simulink model "Part_f"  (R2016a)
settings: Solver=VariableStepAuto  StartTime=0.0  StopTime=10.0  RelTol=1e-3
values from neighbouring files (symbols this model uses):
  A = [1,0.00958419619475136,0.0104077383156783,0;0,0.880217654134450,2.02956823954280,0;0,-0.102406711940655,0.862350586928406,0;1,0.00958419619475136,0.0104077383156783,1]    [Project_2.m]
  B = [0.0388811995595289;11.5416986681227;10.5268226869341;0.0388811995595289]    [Project_2.m]
  C = [0,0,0,1]    [Project_2.m]
  L = acker(A',C',PO)'    [Project_2.m]
  x0 = [.2;0;0;0]    [Project_2.m]
settings Model: Creator=ACER  LastModifiedBy=ACER

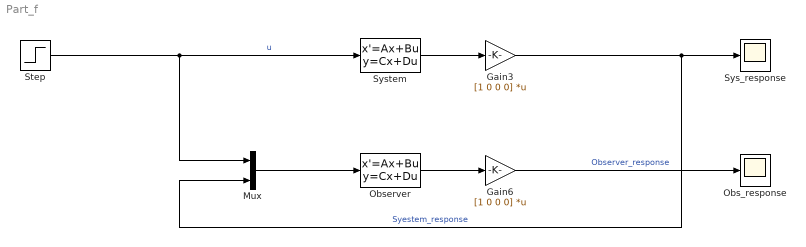
== system Part_f ==
  Gain3 : Gain  Gain=[1 0 0 0]  Multiplication=Matrix(K*u)
  Gain6 : Gain  Gain=[1 0 0 0]  Multiplication=Matrix(K*u)
  Mux : Mux  Inputs=2
  Obs_response : Scope
  Observer : StateSpace  A=A-L*C  B=[B L]  C=eye(4)  D=[0 0;0 0;0 0;0 0]  X0=0
  Step : Step  Time=0  SampleTime=0
  Sys_response : Scope
  System : StateSpace  A=A  B=B  C=eye(4)  D=[0;0;0;0]  X0=x0
  wires:
  System/1 -> Gain3/1
  Gain3/1 -> Mux/2, Sys_response/1  "Syestem_response"
  Observer/1 -> Gain6/1
  Gain6/1 -> Obs_response/1  "Observer_response"
  Step/1 -> Mux/1, System/1  "u"
  Mux/1 -> Observer/1
